simulink model "vdn7_planning_trace_MPC"  (R2022b)
settings: Solver=ode45  StartTime=0.0  StopTime=40  FixedStep=0.01  RelTol=1e-3  EnableMultiTasking=on
libraries: Solver_SF x1
settings Model: Creator=xuwei  LastModifiedBy=wyx
settings SolverCC: AlgebraicLoopSolver=TrustRegion
settings DataIOCC: LimitDataPoints=on  SaveFormat=Array  SignalLoggingSaveFormat=ModelDataLogs  ReturnWorkspaceOutputs=off
settings OptimizationCC: ExpressionDepthLimit=2147483647  LifeSpan=inf
settings DebuggingCC: UnderspecifiedInitializationDetection=Classic  MergeDetectMultiDrivingBlocksExec=none  SolverPrmCheckMsg=warning  FcnCallInpInsideContextMsg=warning  UnconnectedInputMsg=warning  UnconnectedOutputMsg=warning  UnconnectedLineMsg=warning  StateNameClashWarn=warning  SFUnexpectedBacktrackingDiag=warning  SFNoUnconditionalDefaultTransitionDiag=warning  SFExecutionAtInitializationDiag=none  SFMachineParentedDataDiag=warning  ArithmeticOperatorsInVariantConditions=warning
settings HardwareCC: ProdBitPerPointer=32  ProdBitPerSizeT=32  ProdBitPerPtrDiffT=32  ProdLargestAtomicFloat=None  ProdIntDivRoundTo=Undefined  ProdEndianess=Unspecified  ProdWordSize=32  ProdHWDeviceType=32-bit Generic
settings ModelReferenceCC: PropagateSignalLabelsOutOfModel=off
settings SFSimCC: SimUseLocalCustomCode=off  CustomCodeUndefinedFunction=UseInterfaceOnly
settings RTWCC: RTWUseLocalCustomCode=off
settings CodeAppCC: StateflowObjectComments=on
settings GRTTargetCC: TargetLangStandard=C89/C90 (ANSI)  CombineOutputUpdateFcns=off  GRTInterface=on
settings ConfigComp: CovMetricSettings=dw  CovSaveCumulativeToWorkspaceVar=on  CovSaveSingleToWorkspaceVar=on  CovExternalEMLEnable=off
settings SimscapeCC: SimscapeNormalizeSystem=off
settings ConfigurationSet: Description=SimMechanics 2G

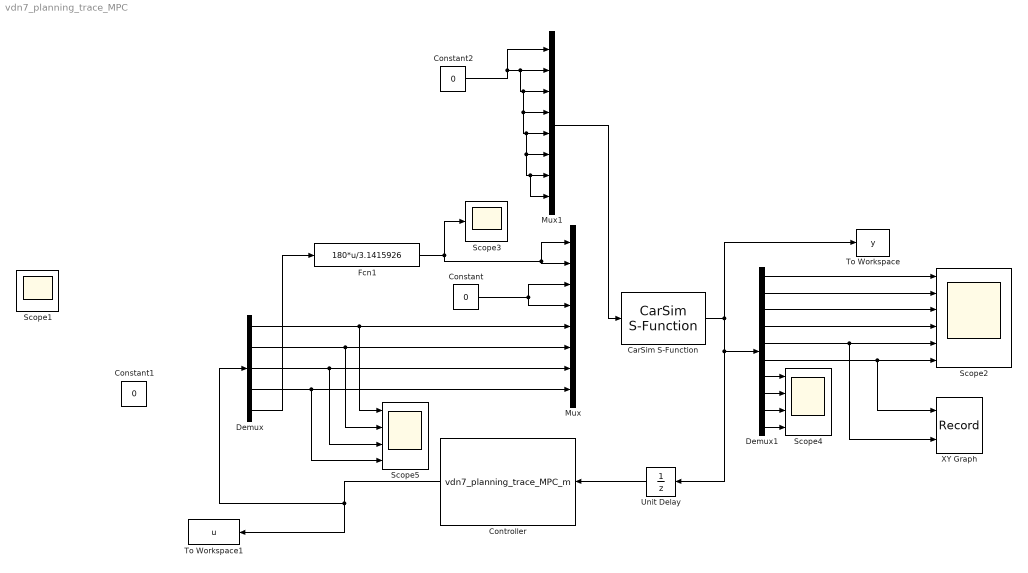
== system vdn7_planning_trace_MPC ==
  CarSim S-Function : Solver_SF/CarSim S-Function  Priority=1  SIMFILE=simfile.sim
  Constant : Constant  Value=0
  Constant1 : Constant  Value=0
  Constant2 : Constant  Value=0
  Controller : S-Function  FunctionName=vdn7_planning_trace_MPC_m  SFunctionDeploymentMode=off  EnableBusSupport=off
  Demux : Demux  Outputs=5
  Demux1 : Demux  Outputs=10
  Fcn1 : Fcn  Expr=180*u/3.1415926
  Mux : Mux  Inputs=8
  Mux1 : Mux  Inputs=8
  Scope1 : Scope  NumInputPorts=2
  Scope2 : Scope  NumInputPorts=6
  Scope3 : Scope
  Scope4 : Scope  NumInputPorts=4
  Scope5 : Scope  NumInputPorts=4
  To Workspace : ToWorkspace  VariableName=y  SaveFormat=Structure  SampleTime=-1
  To Workspace1 : ToWorkspace  VariableName=u  SaveFormat=Structure  SampleTime=-1
  Unit Delay : UnitDelay  SampleTime=-1  HasFrameUpgradeWarning=on
  XY Graph : Record  FileSettingsInternal="{\"entries\":[{\"content\":{\"excelSettings\":{\"content\":{},\"type\":\"Streamout.ExcelSettings\"}},\"type\":\"Streamout.FileSettingStorage\",\"uuid\":\"c2788ee9-f7c8-4a3f-b405-aa862d253017\"}],\"packageUris\":[\"http://schema.mathworks.com/mf0/streamout_blocks/R2020a\"],\"version\":\"1.0\"}"  Layout=[1 1]  SignalsInternal="{\"entries\":[{\"content\":{\"signals\":[{\"content\":{\"blockPath\":[\"vdn7_planning_trace_MPC/XY Graph\"],\"channel\":[],\"dimensions\":[1],\"domain\":\"vdn7_planning_trace_MPC/XY Graph\",\"lineColor\":\"#77ac30\",\"plots\":[],\"port\":1,\"sid\":[\"\"],\"signalID\":1769,\"signalName\":\"Demux1:6\"},\"type\":\"RecordBlkView.Signal\",\"uuid\":\"091db848-1eaf-4cba-b437-8a6da7a9f485\"},{\"content\":{\"blockPath\":[\"vdn7_planning_trace_MPC/XY Graph\"],\"channel\":[],\"dimensions\":[1],\"domain\":\"vdn7_planning_trace_MPC/XY Graph\",\"lineColor\":\"#4dbeee\",\"plots\":[],\"port\":2,\"sid\":[\"\"],\"signalID\":1773,\"signalName\":\"Demux1:5\"},\"type\":\"RecordBlkView.Signal\",\"uuid\":\"375cfcb7-a985-4274-a5b4-af0e1c0201eb\"}]},\"type\":\"RecordBlkView.InputSignals\",\"uuid\":\"533b529a-9ec1-431c-a1a7-1cf404045618\"}],\"packageUris\":[\"http://schema.mathworks.com/mf0/streamout_blocks/R2020a\"],\"version\":\"1.0\"}"  VisualizationBindings="{\"xyplotplugin\":{\"info\":[{\"series\":[],\"subplotID\":1}]}}"  CompatibilityTag=XY  st=-1
  wires:
  CarSim S-Function/1 -> Demux1/1, Unit Delay/1, To Workspace/1
  Demux1/1 -> Scope2/1
  Demux1/2 -> Scope2/2
  Demux1/3 -> Scope2/3
  Demux1/5 -> XY Graph/2, Scope2/5
  Demux1/6 -> XY Graph/1, Scope2/6
  Constant/1 -> Mux/3, Mux/4
  Fcn1/1 -> Mux/2, Mux/1, Scope3/1
  Controller/1 -> To Workspace1/1, Demux/1
  Demux1/4 -> Scope2/4
  Demux/1 -> Scope5/1, Mux/5
  Demux/2 -> Scope5/2, Mux/6
  Demux/3 -> Scope5/3, Mux/7
  Demux/4 -> Scope5/4, Mux/8
  Demux/5 -> Fcn1/1
  Demux1/7 -> Scope4/1
  Demux1/8 -> Scope4/2
  Demux1/9 -> Scope4/3
  Demux1/10 -> Scope4/4
  Mux1/1 -> CarSim S-Function/1
  Constant2/1 -> Mux1/8, Mux1/7, Mux1/6, Mux1/5, Mux1/4, Mux1/3, Mux1/2, Mux1/1
  Unit Delay/1 -> Controller/1
